simulink model "electrical"  (R2024a)
settings: Solver=VariableStepAuto  StartTime=0.0  StopTime=10.0  RelTol=1e-3
libraries: spsSeriesRLCBranchLib x4, simulink x2, spsDCVoltageSourceLib x1, spsVoltageMeasurementLib x1, sps_lib x1
settings Model: Creator=mostafa kamal  LastModifiedBy=mostafa kamal

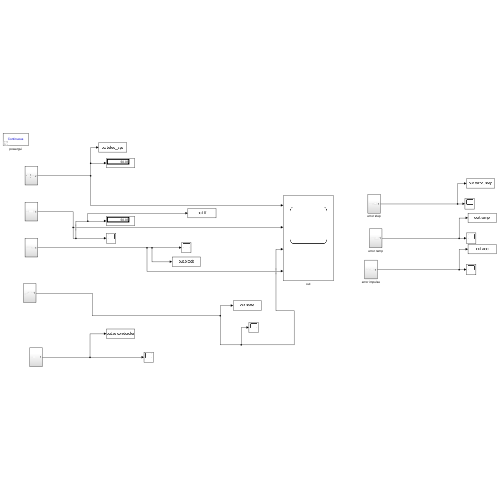
[thumbnail: Simulink's stored preview of the top-level diagram]
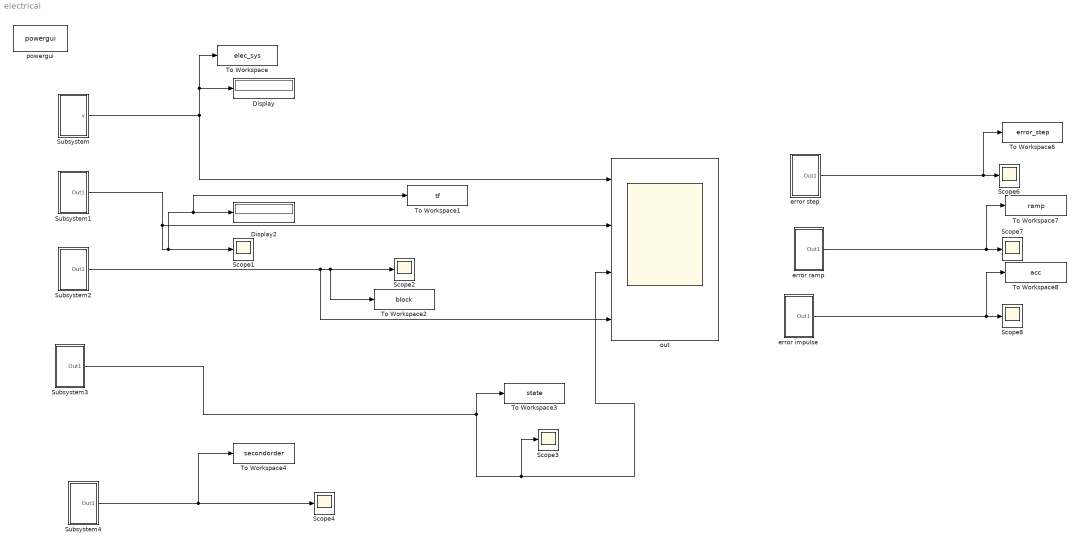
== system electrical ==
  Display : Display
  Display2 : Display
  Scope{1..4,6..8} (7 alike) : Scope
  Subsystem : Subsystem
  Subsystem1 : Subsystem
  Subsystem2 : Subsystem
  Subsystem3 : Subsystem
  Subsystem4 : Subsystem
  To Workspace : ToWorkspace  VariableName=elec_sys  SaveFormat=Timeseries  SampleTime=-1
  To Workspace1 : ToWorkspace  VariableName=tf  SaveFormat=Timeseries  SampleTime=-1
  To Workspace2 : ToWorkspace  VariableName=block  SaveFormat=Timeseries  SampleTime=-1
  To Workspace3 : ToWorkspace  VariableName=state  SaveFormat=Timeseries  SampleTime=-1
  To Workspace4 : ToWorkspace  VariableName=secondorder  SaveFormat=Timeseries  SampleTime=-1
  To Workspace6 : ToWorkspace  VariableName=error_step  SaveFormat=Timeseries  SampleTime=-1
  To Workspace7 : ToWorkspace  VariableName=ramp  SaveFormat=Timeseries  SampleTime=-1
  To Workspace8 : ToWorkspace  VariableName=acc  SaveFormat=Timeseries  SampleTime=-1
  error impulse : Subsystem
  error ramp : Subsystem
  error step : Subsystem
  out : Scope  NumInputPorts=4
  powergui : sps_lib/powergui  Priority=1  SimulationMode=Continuous  SampleTime=50e-6  frequency=60  Iterations=50  frequencyindice=0  Pbase=100e6  ErrMax=1e-4  UnitsV=kV  UnitsW=MW  buscounter=0  FunctionMessages=off  echomessages=off  EnableUseOfTLC=off  CurrentSourceSwitches=off  DisableSnubberDevices=off  DisableRonSwitches=off  DisableVfSwitches=off  DisplayEquations=off  AutomaticDiscreteSolvers=off  SolverType=Tustin/Backward Euler (TBE)  Interpol=off  ExternalGateDelay=off  methode=off  Ts=100  x0status=blocks  SPID=on  SwTol=0  HookPort=off  NonlinearTolerance=1e-4  nMaxIteration=100  ContinueOnMaxIteration=off  RestoreLinks=warning  ResistiveCurrentMeasurement=off  Frange=[0:2:500]  Ylog=off  Xlog=on  ShowGrid=off  save=off  variable=ZData  structure=0  ZoomFFT=off  StartTime=0.0  cycles=1  DisplayStyle=1  fundamental=60  FreqAxis=off  MaxFrequency=1000  frequencyindicesteady=1  RmsSteady=1  display=off
  wires:
  Subsystem1/1(Out1) -> To Workspace1/1, Display2/1, Scope1/1, out/2
  Subsystem4/1(Out1) -> To Workspace4/1, Scope4/1
  Subsystem/1(v) -> out/1, To Workspace/1, Display/1
  Subsystem2/1(Out1) -> out/4, To Workspace2/1, Scope2/1
  Subsystem3/1(Out1) -> out/3, Scope3/1, To Workspace3/1
  error step/1(Out1) -> Scope6/1, To Workspace6/1
  error ramp/1(Out1) -> To Workspace7/1, Scope7/1
  error impulse/1(Out1) -> Scope8/1, To Workspace8/1

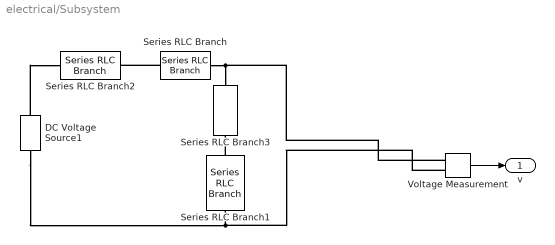
== system electrical/Subsystem ==
  DC Voltage Source1 : spsDCVoltageSourceLib/DC Voltage Source  Amplitude=100  Measurements=None
  Series RLC Branch : spsSeriesRLCBranchLib/Series RLC Branch  LConnTagsString=__new0  RConnTagsString=__new0  BranchType=R  Resistance=1  Inductance=1e-3  SetiL0=off  InitialCurrent=0  Capacitance=1e-6  Setx0=off  InitialVoltage=0  Measurements=None
  Series RLC Branch1 : spsSeriesRLCBranchLib/Series RLC Branch  LConnTagsString=__new0  RConnTagsString=__new0  BranchType=L  Resistance=1  Inductance=1  SetiL0=on  InitialCurrent=0  Capacitance=1e-6  Setx0=off  InitialVoltage=0  Measurements=None
  Series RLC Branch2 : spsSeriesRLCBranchLib/Series RLC Branch  LConnTagsString=__new0  RConnTagsString=__new0  BranchType=C  Resistance=1  Inductance=1e-3  SetiL0=off  InitialCurrent=0  Capacitance=1  Setx0=on  InitialVoltage=0  Measurements=None
  Series RLC Branch3 : spsSeriesRLCBranchLib/Series RLC Branch  LConnTagsString=__new0  RConnTagsString=__new0  BranchType=C  Resistance=1  Inductance=1e-3  SetiL0=off  InitialCurrent=0  Capacitance=1  Setx0=on  InitialVoltage=0  Measurements=None
  Voltage Measurement : spsVoltageMeasurementLib/Voltage Measurement  PhasorSimulation=off  OutputType=Complex  PSBequivalent=0
  v : Outport
  wires:
  Voltage Measurement/1 -> v/1
  connections:
  Series RLC Branch1/LConn1 -- Series RLC Branch3/RConn1
  DC Voltage Source1/RConn1 -- Series RLC Branch2/LConn1
  Voltage Measurement/LConn2 -- DC Voltage Source1/LConn1 -- Series RLC Branch1/RConn1
  Series RLC Branch/RConn1 -- Series RLC Branch3/LConn1 -- Voltage Measurement/LConn1
  Series RLC Branch/LConn1 -- Series RLC Branch2/RConn1

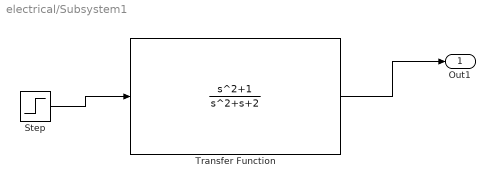
== system electrical/Subsystem1 ==
  Step : Step  Time=0  After=100  SampleTime=0
  Transfer Function : TransferFcn  Numerator=[1 0 1]  Denominator=[1 1 2]
  Out1 : Outport
  wires:
  Step/1 -> Transfer Function/1
  Transfer Function/1 -> Out1/1

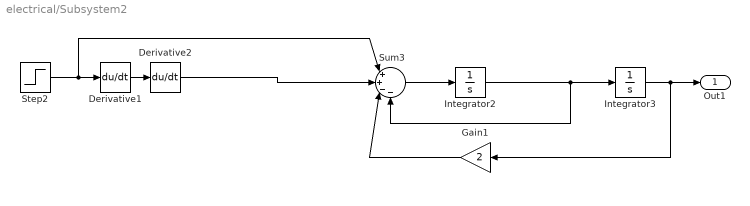
== system electrical/Subsystem2 ==
  Derivative1 : Derivative
  Derivative2 : Derivative
  Gain1 : Gain  Gain=2
  Integrator2 : Integrator
  Integrator3 : Integrator
  Step2 : Step  Time=0  After=100  SampleTime=0
  Sum3 : Sum  Inputs=|++--
  Out1 : Outport
  wires:
  Derivative2/1 -> Sum3/2
  Sum3/1 -> Integrator2/1
  Integrator3/1 -> Out1/1, Gain1/1
  Gain1/1 -> Sum3/3
  Derivative1/1 -> Derivative2/1
  Step2/1 -> Sum3/1, Derivative1/1
  Integrator2/1 -> Sum3/4, Integrator3/1

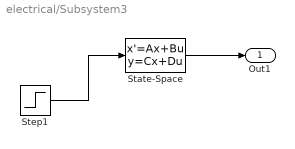
== system electrical/Subsystem3 ==
  State-Space : StateSpace  A=[0 1;-2 -1]  B=[0;1]  C=[-1 -1]  D=[1]  InitialCondition=0
  Step1 : Step  Time=0  After=100  SampleTime=0
  Out1 : Outport
  wires:
  Step1/1 -> State-Space/1
  State-Space/1 -> Out1/1

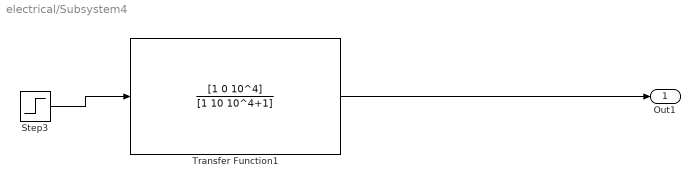
== system electrical/Subsystem4 ==
  Step3 : Step  Time=0  After=100  SampleTime=0
  Transfer Function1 : TransferFcn  Numerator=[1 0 10^4]  Denominator=[1 10 10^4+1]
  Out1 : Outport
  wires:
  Step3/1 -> Transfer Function1/1
  Transfer Function1/1 -> Out1/1

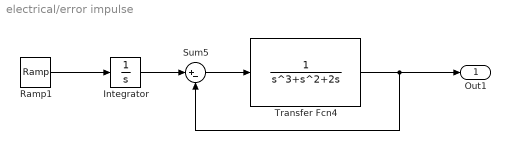
== system electrical/error impulse ==
  Integrator : Integrator
  Ramp1 : simulink/Sources/Ramp  slope=1  start=0  InitialOutput=0
  Sum5 : Sum  Inputs=|+-
  Transfer Fcn4 : TransferFcn  Denominator=[1 1 2 0]
  Out1 : Outport
  wires:
  Ramp1/1 -> Integrator/1
  Transfer Fcn4/1 -> Out1/1, Sum5/2
  Sum5/1 -> Transfer Fcn4/1
  Integrator/1 -> Sum5/1

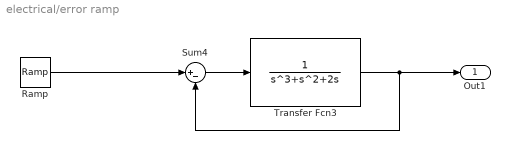
== system electrical/error ramp ==
  Ramp : simulink/Sources/Ramp  slope=1  start=0  InitialOutput=0
  Sum4 : Sum  Inputs=|+-
  Transfer Fcn3 : TransferFcn  Denominator=[1 1 2 0]
  Out1 : Outport
  wires:
  Ramp/1 -> Sum4/1
  Sum4/1 -> Transfer Fcn3/1
  Transfer Fcn3/1 -> Out1/1, Sum4/2

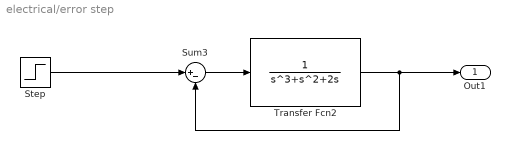
== system electrical/error step ==
  Step : Step  SampleTime=0
  Sum3 : Sum  Inputs=|+-
  Transfer Fcn2 : TransferFcn  Denominator=[1 1 2 0]
  Out1 : Outport
  wires:
  Transfer Fcn2/1 -> Out1/1, Sum3/2
  Sum3/1 -> Transfer Fcn2/1
  Step/1 -> Sum3/1
